simulink library "halout"  (R2021b)
settings: Solver=VariableStepAuto  StartTime=0.0  StopTime=10.0  RelTol=1e-3
undefined symbols (not defined in the file): C_TASK_5MS_S, FALSE, KHAL_CAN1FDAPS3E2E_flg, KHAL_CAN1FDAPS3TxReq_flg, KHAL_CAN1FDVCU2E2E_flg, KHAL_CAN1FDVCU2TxReq_flg, KHAL_CAN1FDVCU3E2E_flg, KHAL_CAN1FDVCU3TxReq_flg, KHAL_CAN1TxReq_flg, KHAL_CAN2TxReq_flg, KHAL_CAN3FDVCU1TxReq_flg, KHAL_CAN3FDVCU2E2E_flg, KHAL_CAN3FDVCU2TxReq_flg, KHAL_CAN3TxReq_flg, KHAL_CAN4FDVCU1E2E_flg, KHAL_CAN4FDVCU1TxReq_flg, KHAL_CAN4TxReq_flg, KHAL_CAN5TxReq_flg, ONE_INT, TRUE, ZERO_INT
libraries: FVT_lib x383, simulink x179
(part 15 of 20)

== system halout/HAL_OUT/CAN2/FD_VCU0_0x1F0/SysAllowReadySta ==
  SysAllowReadySta : Inport
  Data Type Conversion : DataTypeConversion  OutDataTypeStr=uint8  RndMeth=Round
  CAN2_SysAllowReadySta : Outport
  wires:
  Data Type Conversion/1 -> CAN2_SysAllowReadySta/1
  SysAllowReadySta/1 -> Data Type Conversion/1

== system halout/HAL_OUT/CAN2/FD_VCU0_0x1F0/SysPwrSta ==
  SysPwrSta : Inport
  Data Type Conversion : DataTypeConversion  OutDataTypeStr=uint8  RndMeth=Round
  CAN2_SysPwrSta : Outport
  wires:
  Data Type Conversion/1 -> CAN2_SysPwrSta/1
  SysPwrSta/1 -> Data Type Conversion/1

== system halout/HAL_OUT/CAN2/FD_VCU0_0x1F0/TCountSta ==
  TCountSta : Inport
  Data Type Conversion : DataTypeConversion  OutDataTypeStr=uint8  RndMeth=Round
  CAN2_TCountSta : Outport
  wires:
  Data Type Conversion/1 -> CAN2_TCountSta/1
  TCountSta/1 -> Data Type Conversion/1

== system halout/HAL_OUT/CAN2/FD_VCU0_0x1F0/TimerAllowSleep ==
  TimerAllowSleep : Inport
  Data Type Conversion : DataTypeConversion  OutDataTypeStr=uint8  RndMeth=Round
  CAN2_TimerAllowSleep : Outport
  wires:
  Data Type Conversion/1 -> CAN2_TimerAllowSleep/1
  TimerAllowSleep/1 -> Data Type Conversion/1

== system halout/HAL_OUT/CAN2/FD_VCU0_0x1F0/VCUBrkSWSta ==
  VCUBrkSWSta : Inport
  Data Type Conversion : DataTypeConversion  OutDataTypeStr=uint8  RndMeth=Round
  CAN2_VCUBrkSWSta : Outport
  wires:
  Data Type Conversion/1 -> CAN2_VCUBrkSWSta/1
  VCUBrkSWSta/1 -> Data Type Conversion/1

== system halout/HAL_OUT/CAN2/FD_VCU0_0x1F0/VCUFLDoorSta ==
  VCUFLDoorSta : Inport
  Data Type Conversion : DataTypeConversion  OutDataTypeStr=uint8  RndMeth=Round
  CAN2_VCUFLDoorSta : Outport
  wires:
  Data Type Conversion/1 -> CAN2_VCUFLDoorSta/1
  VCUFLDoorSta/1 -> Data Type Conversion/1

== system halout/HAL_OUT/CAN2/FD_VCU0_0x1F0/VCUFRDoorSta ==
  VCUFRDoorSta : Inport
  Data Type Conversion : DataTypeConversion  OutDataTypeStr=uint8  RndMeth=Round
  CAN2_VCUFRDoorSta : Outport
  wires:
  Data Type Conversion/1 -> CAN2_VCUFRDoorSta/1
  VCUFRDoorSta/1 -> Data Type Conversion/1

== system halout/HAL_OUT/CAN2/FD_VCU0_0x1F0/VCUHoodSWSta ==
  VCUHoodSWSta : Inport
  Data Type Conversion : DataTypeConversion  OutDataTypeStr=uint8  RndMeth=Round
  CAN2_VCUHoodSWSta : Outport
  wires:
  Data Type Conversion/1 -> CAN2_VCUHoodSWSta/1
  VCUHoodSWSta/1 -> Data Type Conversion/1

== system halout/HAL_OUT/CAN2/FD_VCU0_0x1F0/VCURLDoorSta ==
  VCURLDoorSta : Inport
  Data Type Conversion : DataTypeConversion  OutDataTypeStr=uint8  RndMeth=Round
  CAN2_VCURLDoorSta : Outport
  wires:
  Data Type Conversion/1 -> CAN2_VCURLDoorSta/1
  VCURLDoorSta/1 -> Data Type Conversion/1

== system halout/HAL_OUT/CAN2/FD_VCU0_0x1F0/VCURRDoorSta ==
  VCURRDoorSta : Inport
  Data Type Conversion : DataTypeConversion  OutDataTypeStr=uint8  RndMeth=Round
  CAN2_VCURRDoorSta : Outport
  wires:
  Data Type Conversion/1 -> CAN2_VCURRDoorSta/1
  VCURRDoorSta/1 -> Data Type Conversion/1

== system halout/HAL_OUT/CAN2/FD_VCU0_0x1F0/VCUTailgateSWSta ==
  VCUTailgateSWSta : Inport
  Data Type Conversion : DataTypeConversion  OutDataTypeStr=uint8  RndMeth=Round
  CAN2_VCUTailgateSWSta : Outport
  wires:
  Data Type Conversion/1 -> CAN2_VCUTailgateSWSta/1
  VCUTailgateSWSta/1 -> Data Type Conversion/1

== system halout/HAL_OUT/CAN2/FD_VCU0_0x1F0/VehHVPwrAvail4THCM ==
  VehHVPwrAvail4THCM : Inport
  Data Type Conversion : DataTypeConversion  OutDataTypeStr=uint8  RndMeth=Round
  convert_out : FVT_lib/hal/convert_out  gain=50  offset=0
  CAN2_VehHVPwrAvail4THCM : Outport
  wires:
  Data Type Conversion/1 -> CAN2_VehHVPwrAvail4THCM/1
  convert_out/1 -> Data Type Conversion/1
  VehHVPwrAvail4THCM/1 -> convert_out/1

== system halout/HAL_OUT/CAN2/FD_VCU1_0x116/ActiveDischReq ==
  ActiveDischReq : Inport
  Data Type Conversion : DataTypeConversion  OutDataTypeStr=uint8  RndMeth=Round
  CAN2_ActiveDischReq : Outport
  wires:
  Data Type Conversion/1 -> CAN2_ActiveDischReq/1
  ActiveDischReq/1 -> Data Type Conversion/1

== system halout/HAL_OUT/CAN2/FD_VCU1_0x116/CCCrlSta ==
  CCCrlSta : Inport
  Data Type Conversion : DataTypeConversion  OutDataTypeStr=uint8  RndMeth=Round
  CAN2_CC_Crl_Sta : Outport
  wires:
  Data Type Conversion/1 -> CAN2_CC_Crl_Sta/1
  CCCrlSta/1 -> Data Type Conversion/1

== system halout/HAL_OUT/CAN2/FD_VCU1_0x116/CSVCU1CAN2 ==
  CSVCU1CAN2 : Inport
  Data Type Conversion : DataTypeConversion  OutDataTypeStr=uint8  RndMeth=Round
  CAN2_CS_VCU1_CAN2 : Outport
  wires:
  Data Type Conversion/1 -> CAN2_CS_VCU1_CAN2/1
  CSVCU1CAN2/1 -> Data Type Conversion/1

== system halout/HAL_OUT/CAN2/FD_VCU1_0x116/CoastDwModeStaChk ==
  CoastDwModeStaChk : Inport
  Data Type Conversion : DataTypeConversion  OutDataTypeStr=uint8  RndMeth=Round
  CAN2_CoastDwModeStaChk : Outport
  wires:
  Data Type Conversion/1 -> CAN2_CoastDwModeStaChk/1
  CoastDwModeStaChk/1 -> Data Type Conversion/1

== system halout/HAL_OUT/CAN2/FD_VCU1_0x116/CreepSWSta ==
  CreepSWSta : Inport
  Data Type Conversion : DataTypeConversion  OutDataTypeStr=uint8  RndMeth=Round
  CAN2_CreepSW_Sta : Outport
  wires:
  Data Type Conversion/1 -> CAN2_CreepSW_Sta/1
  CreepSWSta/1 -> Data Type Conversion/1

== system halout/HAL_OUT/CAN2/FD_VCU1_0x116/DCDCEnaReq ==
  DCDCEnaReq : Inport
  Data Type Conversion : DataTypeConversion  OutDataTypeStr=uint8  RndMeth=Round
  CAN2_DCDCEnaReq : Outport
  wires:
  Data Type Conversion/1 -> CAN2_DCDCEnaReq/1
  DCDCEnaReq/1 -> Data Type Conversion/1

== system halout/HAL_OUT/CAN2/FD_VCU1_0x116/DCDCVoltSetpoint ==
  DCDCVoltSetpoint : Inport
  Data Type Conversion : DataTypeConversion  OutDataTypeStr=uint8  RndMeth=Round
  convert_out : FVT_lib/hal/convert_out  gain=0.0235  offset=12
  CAN2_DCDCVoltSetpoint : Outport
  wires:
  Data Type Conversion/1 -> CAN2_DCDCVoltSetpoint/1
  convert_out/1 -> Data Type Conversion/1
  DCDCVoltSetpoint/1 -> convert_out/1

== system halout/HAL_OUT/CAN2/FD_VCU1_0x116/DemoModeStaChk ==
  DemoModeStaChk : Inport
  Data Type Conversion : DataTypeConversion  OutDataTypeStr=uint8  RndMeth=Round
  CAN2_DemoModeStaChk : Outport
  wires:
  Data Type Conversion/1 -> CAN2_DemoModeStaChk/1
  DemoModeStaChk/1 -> Data Type Conversion/1

== system halout/HAL_OUT/CAN2/FD_VCU1_0x116/DisengagePFail ==
  DisengagePFail : Inport
  Data Type Conversion : DataTypeConversion  OutDataTypeStr=uint8  RndMeth=Round
  CAN2_DisengageP_Fail : Outport
  wires:
  Data Type Conversion/1 -> CAN2_DisengageP_Fail/1
  DisengagePFail/1 -> Data Type Conversion/1

== system halout/HAL_OUT/CAN2/FD_VCU1_0x116/DrSeatSta ==
  DrSeatSta : Inport
  Data Type Conversion : DataTypeConversion  OutDataTypeStr=uint8  RndMeth=Round
  CAN2_Dr_SeatSta : Outport
  wires:
  Data Type Conversion/1 -> CAN2_Dr_SeatSta/1
  DrSeatSta/1 -> Data Type Conversion/1

== system halout/HAL_OUT/CAN2/FD_VCU1_0x116/DynoModeStaChk ==
  DynoModeStaChk : Inport
  Data Type Conversion : DataTypeConversion  OutDataTypeStr=uint8  RndMeth=Round
  CAN2_DynoModeStaChk : Outport
  wires:
  Data Type Conversion/1 -> CAN2_DynoModeStaChk/1
  DynoModeStaChk/1 -> Data Type Conversion/1

== system halout/HAL_OUT/CAN2/FD_VCU1_0x116/EngagePFail ==
  EngagePFail : Inport
  Data Type Conversion : DataTypeConversion  OutDataTypeStr=uint8  RndMeth=Round
  CAN2_EngageP_Fail : Outport
  wires:
  Data Type Conversion/1 -> CAN2_EngageP_Fail/1
  EngagePFail/1 -> Data Type Conversion/1

== system halout/HAL_OUT/CAN2/FD_VCU1_0x116/FDCVCUPwrSaveReqCmd ==
  FDCVCUPwrSaveReqCmd : Inport
  Data Type Conversion : DataTypeConversion  OutDataTypeStr=uint8  RndMeth=Round
  CAN2_FDC_VCU_PwrSaveReq_Cmd : Outport
  wires:
  Data Type Conversion/1 -> CAN2_FDC_VCU_PwrSaveReq_Cmd/1
  FDCVCUPwrSaveReqCmd/1 -> Data Type Conversion/1

== system halout/HAL_OUT/CAN2/FD_VCU1_0x116/FalseNPreventSta ==
  FalseNPreventSta : Inport
  Data Type Conversion : DataTypeConversion  OutDataTypeStr=uint8  RndMeth=Round
  CAN2_FalseNPrevent_Sta : Outport
  wires:
  Data Type Conversion/1 -> CAN2_FalseNPrevent_Sta/1
  FalseNPreventSta/1 -> Data Type Conversion/1

== system halout/HAL_OUT/CAN2/FD_VCU1_0x116/FrActvDmpDisabReq ==
  FrActvDmpDisabReq : Inport
  Data Type Conversion : DataTypeConversion  OutDataTypeStr=uint8  RndMeth=Round
  CAN2_Fr_ActvDmpDisabReq : Outport
  wires:
  Data Type Conversion/1 -> CAN2_Fr_ActvDmpDisabReq/1
  FrActvDmpDisabReq/1 -> Data Type Conversion/1

== system halout/HAL_OUT/CAN2/FD_VCU1_0x116/FrMCUEnaReq ==
  FrMCUEnaReq : Inport
  Data Type Conversion : DataTypeConversion  OutDataTypeStr=uint8  RndMeth=Round
  CAN2_Fr_MCUEnaReq : Outport
  wires:
  Data Type Conversion/1 -> CAN2_Fr_MCUEnaReq/1
  FrMCUEnaReq/1 -> Data Type Conversion/1

== system halout/HAL_OUT/CAN2/FD_VCU1_0x116/HVBatCnctReq ==
  HVBatCnctReq : Inport
  Data Type Conversion : DataTypeConversion  OutDataTypeStr=uint8  RndMeth=Round
  CAN2_HVBatCnctReq : Outport
  wires:
  Data Type Conversion/1 -> CAN2_HVBatCnctReq/1
  HVBatCnctReq/1 -> Data Type Conversion/1

== system halout/HAL_OUT/CAN2/FD_VCU1_0x116/HVSysReadyToCharge ==
  HVSysReadyToCharge : Inport
  Data Type Conversion : DataTypeConversion  OutDataTypeStr=uint8  RndMeth=Round
  CAN2_HVSysReadyToCharge : Outport
  wires:
  Data Type Conversion/1 -> CAN2_HVSysReadyToCharge/1
  HVSysReadyToCharge/1 -> Data Type Conversion/1

== system halout/HAL_OUT/CAN2/FD_VCU1_0x116/LVChrgFuncStaChk ==
  LVChrgFuncStaChk : Inport
  Data Type Conversion : DataTypeConversion  OutDataTypeStr=uint8  RndMeth=Round
  CAN2_LVChrgFuncStaChk : Outport
  wires:
  Data Type Conversion/1 -> CAN2_LVChrgFuncStaChk/1
  LVChrgFuncStaChk/1 -> Data Type Conversion/1

== system halout/HAL_OUT/CAN2/FD_VCU1_0x116/MSACrlSta ==
  MSACrlSta : Inport
  Data Type Conversion : DataTypeConversion  OutDataTypeStr=uint8  RndMeth=Round
  CAN2_MSA_Crl_Sta : Outport
  wires:
  Data Type Conversion/1 -> CAN2_MSA_Crl_Sta/1
  MSACrlSta/1 -> Data Type Conversion/1

== system halout/HAL_OUT/CAN2/FD_VCU1_0x116/PrkReq ==
  PrkReq : Inport
  Data Type Conversion : DataTypeConversion  OutDataTypeStr=uint8  RndMeth=Round
  CAN2_PrkReq : Outport
  wires:
  Data Type Conversion/1 -> CAN2_PrkReq/1
  PrkReq/1 -> Data Type Conversion/1

== system halout/HAL_OUT/CAN2/FD_VCU1_0x116/PwrSta ==
  PwrSta : Inport
  Data Type Conversion : DataTypeConversion  OutDataTypeStr=uint8  RndMeth=Round
  CAN2_PwrSta : Outport
  wires:
  Data Type Conversion/1 -> CAN2_PwrSta/1
  PwrSta/1 -> Data Type Conversion/1

== system halout/HAL_OUT/CAN2/FD_VCU1_0x116/RCVCU1CAN2 ==
  RCVCU1CAN2 : Inport
  Data Type Conversion : DataTypeConversion  OutDataTypeStr=uint8  RndMeth=Round
  CAN2_RC_VCU1_CAN2 : Outport
  wires:
  Data Type Conversion/1 -> CAN2_RC_VCU1_CAN2/1
  RCVCU1CAN2/1 -> Data Type Conversion/1

== system halout/HAL_OUT/CAN2/FD_VCU1_0x116/RrActvDmpDisabReq ==
  RrActvDmpDisabReq : Inport
  Data Type Conversion : DataTypeConversion  OutDataTypeStr=uint8  RndMeth=Round
  CAN2_Rr_ActvDmpDisabReq : Outport
  wires:
  Data Type Conversion/1 -> CAN2_Rr_ActvDmpDisabReq/1
  RrActvDmpDisabReq/1 -> Data Type Conversion/1

== system halout/HAL_OUT/CAN2/FD_VCU1_0x116/RrMCUEnaReq ==
  RrMCUEnaReq : Inport
  Data Type Conversion : DataTypeConversion  OutDataTypeStr=uint8  RndMeth=Round
  CAN2_Rr_MCUEnaReq : Outport
  wires:
  Data Type Conversion/1 -> CAN2_Rr_MCUEnaReq/1
  RrMCUEnaReq/1 -> Data Type Conversion/1

== system halout/HAL_OUT/CAN2/FD_VCU1_0x116/ShiftGearPosn ==
  ShiftGearPosn : Inport
  Data Type Conversion : DataTypeConversion  OutDataTypeStr=uint8  RndMeth=Round
  CAN2_ShiftGearPosn : Outport
  wires:
  Data Type Conversion/1 -> CAN2_ShiftGearPosn/1
  ShiftGearPosn/1 -> Data Type Conversion/1

== system halout/HAL_OUT/CAN2/FD_VCU1_0x116/VCUOPDHold ==
  VCUOPDHold : Inport
  Data Type Conversion : DataTypeConversion  OutDataTypeStr=uint8  RndMeth=Round
  CAN2_VCU_OPDHold : Outport
  wires:
  Data Type Conversion/1 -> CAN2_VCU_OPDHold/1
  VCUOPDHold/1 -> Data Type Conversion/1

== system halout/HAL_OUT/CAN2/FD_VCU1_0x116/XWDMode ==
  XWDMode : Inport
  Data Type Conversion : DataTypeConversion  OutDataTypeStr=uint8  RndMeth=Round
  CAN2_XWDMode : Outport
  wires:
  Data Type Conversion/1 -> CAN2_XWDMode/1
  XWDMode/1 -> Data Type Conversion/1

== system halout/HAL_OUT/CAN2/FD_VCU2_0x154/ACCCtrlAvail ==
  ACCCtrlAvail : Inport
  Data Type Conversion : DataTypeConversion  OutDataTypeStr=uint8  RndMeth=Round
  CAN2_ACC_CtrlAvail : Outport
  wires:
  Data Type Conversion/1 -> CAN2_ACC_CtrlAvail/1
  ACCCtrlAvail/1 -> Data Type Conversion/1

== system halout/HAL_OUT/CAN2/FD_VCU2_0x154/AccPedalOverride ==
  AccPedalOverride : Inport
  Data Type Conversion : DataTypeConversion  OutDataTypeStr=uint8  RndMeth=Round
  CAN2_AccPedal_Override : Outport
  wires:
  Data Type Conversion/1 -> CAN2_AccPedal_Override/1
  AccPedalOverride/1 -> Data Type Conversion/1

== system halout/HAL_OUT/CAN2/FD_VCU2_0x154/ActAPSPosn ==
  ActAPSPosn : Inport
  Data Type Conversion : DataTypeConversion  OutDataTypeStr=uint8  RndMeth=Round
  convert_out : FVT_lib/hal/convert_out  gain=0.394  offset=0
  CAN2_ActAPSPosn : Outport
  wires:
  Data Type Conversion/1 -> CAN2_ActAPSPosn/1
  convert_out/1 -> Data Type Conversion/1
  ActAPSPosn/1 -> convert_out/1

== system halout/HAL_OUT/CAN2/FD_VCU2_0x154/CSVCU2CAN1 ==
  CSVCU2CAN1 : Inport
  Data Type Conversion : DataTypeConversion  OutDataTypeStr=uint8  RndMeth=Round
  CAN2_CS_VCU2_CAN1 : Outport
  wires:
  Data Type Conversion/1 -> CAN2_CS_VCU2_CAN1/1
  CSVCU2CAN1/1 -> Data Type Conversion/1

== system halout/HAL_OUT/CAN2/FD_VCU2_0x154/DriverTq ==
  DriverTq : Inport
  Data Type Conversion : DataTypeConversion  OutDataTypeStr=uint16  RndMeth=Round
  convert_out : FVT_lib/hal/convert_out  gain=1  offset=-4300
  CAN2_DriverTq : Outport
  wires:
  Data Type Conversion/1 -> CAN2_DriverTq/1
  convert_out/1 -> Data Type Conversion/1
  DriverTq/1 -> convert_out/1

== system halout/HAL_OUT/CAN2/FD_VCU2_0x154/FrDriverTq ==
  FrDriverTq : Inport
  Data Type Conversion : DataTypeConversion  OutDataTypeStr=uint16  RndMeth=Round
  convert_out : FVT_lib/hal/convert_out  gain=0.5  offset=-5300
  CAN2_Fr_DriverTq : Outport
  wires:
  Data Type Conversion/1 -> CAN2_Fr_DriverTq/1
  convert_out/1 -> Data Type Conversion/1
  FrDriverTq/1 -> convert_out/1

== system halout/HAL_OUT/CAN2/FD_VCU2_0x154/RCVCU2CAN1 ==
  RCVCU2CAN1 : Inport
  Data Type Conversion : DataTypeConversion  OutDataTypeStr=uint8  RndMeth=Round
  CAN2_RC_VCU2_CAN1 : Outport
  wires:
  Data Type Conversion/1 -> CAN2_RC_VCU2_CAN1/1
  RCVCU2CAN1/1 -> Data Type Conversion/1

== system halout/HAL_OUT/CAN2/FD_VCU2_0x154/RrDriverTq ==
  RrDriverTq : Inport
  Data Type Conversion : DataTypeConversion  OutDataTypeStr=uint16  RndMeth=Round
  convert_out : FVT_lib/hal/convert_out  gain=0.5  offset=-5300
  CAN2_Rr_DriverTq : Outport
  wires:
  Data Type Conversion/1 -> CAN2_Rr_DriverTq/1
  convert_out/1 -> Data Type Conversion/1
  RrDriverTq/1 -> convert_out/1

== system halout/HAL_OUT/CAN2/FD_VCU2_0x154/VehActPwr ==
  VehActPwr : Inport
  Data Type Conversion : DataTypeConversion  OutDataTypeStr=uint32  RndMeth=Round
  convert_out : FVT_lib/hal/convert_out  gain=1  offset=-600000
  CAN2_VehActPwr : Outport
  wires:
  Data Type Conversion/1 -> CAN2_VehActPwr/1
  convert_out/1 -> Data Type Conversion/1
  VehActPwr/1 -> convert_out/1

== system halout/HAL_OUT/CAN2/FD_VCU4_0x3C0/EVDriveMode ==
  EVDriveMode : Inport
  Data Type Conversion : DataTypeConversion  OutDataTypeStr=uint8  RndMeth=Round
  CAN2_EVDriveMode : Outport
  wires:
  Data Type Conversion/1 -> CAN2_EVDriveMode/1
  EVDriveMode/1 -> Data Type Conversion/1

== system halout/HAL_OUT/CAN2/FD_VCU4_0x3C0/EngAGSCloseSta ==
  EngAGSCloseSta : Inport
  Data Type Conversion : DataTypeConversion  OutDataTypeStr=uint8  RndMeth=Round
  CAN2_Eng_AGSCloseSta : Outport
  wires:
  Data Type Conversion/1 -> CAN2_Eng_AGSCloseSta/1
  EngAGSCloseSta/1 -> Data Type Conversion/1

== system halout/HAL_OUT/CAN2/FD_VCU4_0x3C0/EngActvDmpDisabSta ==
  EngActvDmpDisabSta : Inport
  Data Type Conversion : DataTypeConversion  OutDataTypeStr=uint8  RndMeth=Round
  CAN2_Eng_ActvDmpDisabSta : Outport
  wires:
  Data Type Conversion/1 -> CAN2_Eng_ActvDmpDisabSta/1
  EngActvDmpDisabSta/1 -> Data Type Conversion/1

== system halout/HAL_OUT/CAN2/FD_VCU4_0x3C0/EngCoastDwSta ==
  EngCoastDwSta : Inport
  Data Type Conversion : DataTypeConversion  OutDataTypeStr=uint8  RndMeth=Round
  CAN2_Eng_CoastDwSta : Outport
  wires:
  Data Type Conversion/1 -> CAN2_Eng_CoastDwSta/1
  EngCoastDwSta/1 -> Data Type Conversion/1

== system halout/HAL_OUT/CAN2/FD_VCU4_0x3C0/EngPwrLockSta ==
  EngPwrLockSta : Inport
  Data Type Conversion : DataTypeConversion  OutDataTypeStr=uint8  RndMeth=Round
  CAN2_Eng_PwrLockSta : Outport
  wires:
  Data Type Conversion/1 -> CAN2_Eng_PwrLockSta/1
  EngPwrLockSta/1 -> Data Type Conversion/1

== system halout/HAL_OUT/CAN2/FD_VCU4_0x3C0/VCUACCErr ==
  VCUACCErr : Inport
  Data Type Conversion : DataTypeConversion  OutDataTypeStr=uint8  RndMeth=Round
  CAN2_VCU_ACCErr : Outport
  wires:
  Data Type Conversion/1 -> CAN2_VCU_ACCErr/1
  VCUACCErr/1 -> Data Type Conversion/1

== system halout/HAL_OUT/CAN2/FD_VCU4_0x3C0/VCUISAErr ==
  VCUISAErr : Inport
  Data Type Conversion : DataTypeConversion  OutDataTypeStr=uint8  RndMeth=Round
  CAN2_VCU_ISAErr : Outport
  wires:
  Data Type Conversion/1 -> CAN2_VCU_ISAErr/1
  VCUISAErr/1 -> Data Type Conversion/1

== system halout/HAL_OUT/CAN2/FD_VCU4_0x3C0/VehMalfunLevel ==
  VehMalfunLevel : Inport
  Data Type Conversion : DataTypeConversion  OutDataTypeStr=uint8  RndMeth=Round
  CAN2_VehMalfunLevel : Outport
  wires:
  Data Type Conversion/1 -> CAN2_VehMalfunLevel/1
  VehMalfunLevel/1 -> Data Type Conversion/1

== system halout/HAL_OUT/CAN2/FD_VCU4_0x3C0/ZoneDRSCPCommErr ==
  ZoneDRSCPCommErr : Inport
  Data Type Conversion : DataTypeConversion  OutDataTypeStr=uint8  RndMeth=Round
  CAN2_ZoneDR_SCP_CommErr : Outport
  wires:
  Data Type Conversion/1 -> CAN2_ZoneDR_SCP_CommErr/1
  ZoneDRSCPCommErr/1 -> Data Type Conversion/1

== system halout/HAL_OUT/CAN2/FD_VCU5_0x245/EDriveSysErrAccPedalErr ==
  EDriveSysErrAccPedalErr : Inport
  Data Type Conversion : DataTypeConversion  OutDataTypeStr=uint8  RndMeth=Round
  CAN2_EDriveSysErr_AccPedalErr : Outport
  wires:
  Data Type Conversion/1 -> CAN2_EDriveSysErr_AccPedalErr/1
  EDriveSysErrAccPedalErr/1 -> Data Type Conversion/1

== system halout/HAL_OUT/CAN2/FD_VCU5_0x245/EDriveSysErrMCUErr ==
  EDriveSysErrMCUErr : Inport
  Data Type Conversion : DataTypeConversion  OutDataTypeStr=uint8  RndMeth=Round
  CAN2_EDriveSysErr_MCUErr : Outport
  wires:
  Data Type Conversion/1 -> CAN2_EDriveSysErr_MCUErr/1
  EDriveSysErrMCUErr/1 -> Data Type Conversion/1

== system halout/HAL_OUT/CAN2/FD_VCU5_0x245/EDriveSysErrShifterErr ==
  EDriveSysErrShifterErr : Inport
  Data Type Conversion : DataTypeConversion  OutDataTypeStr=uint8  RndMeth=Round
  CAN2_EDriveSysErr_ShifterErr : Outport
  wires:
  Data Type Conversion/1 -> CAN2_EDriveSysErr_ShifterErr/1
  EDriveSysErrShifterErr/1 -> Data Type Conversion/1

== system halout/HAL_OUT/CAN2/FD_VCU5_0x245/EDriveSysErrVCUErr ==
  EDriveSysErrVCUErr : Inport
  Data Type Conversion : DataTypeConversion  OutDataTypeStr=uint8  RndMeth=Round
  CAN2_EDriveSysErr_VCUErr : Outport
  wires:
  Data Type Conversion/1 -> CAN2_EDriveSysErr_VCUErr/1
  EDriveSysErrVCUErr/1 -> Data Type Conversion/1

== system halout/HAL_OUT/CAN2/FD_VCU5_0x245/HVSysErrIsolationErr ==
  HVSysErrIsolationErr : Inport
  Data Type Conversion : DataTypeConversion  OutDataTypeStr=uint8  RndMeth=Round
  CAN2_HVSysErr_IsolationErr : Outport
  wires:
  Data Type Conversion/1 -> CAN2_HVSysErr_IsolationErr/1
  HVSysErrIsolationErr/1 -> Data Type Conversion/1

== system halout/HAL_OUT/CAN2/FD_VCU5_0x245/HVSysErrPackErr ==
  HVSysErrPackErr : Inport
  Data Type Conversion : DataTypeConversion  OutDataTypeStr=uint8  RndMeth=Round
  CAN2_HVSysErr_PackErr : Outport
  wires:
  Data Type Conversion/1 -> CAN2_HVSysErr_PackErr/1
  HVSysErrPackErr/1 -> Data Type Conversion/1

== system halout/HAL_OUT/CAN2/FD_VCU5_0x245/HVSysErrRelayErr ==
  HVSysErrRelayErr : Inport
  Data Type Conversion : DataTypeConversion  OutDataTypeStr=uint8  RndMeth=Round
  CAN2_HVSysErr_RelayErr : Outport
  wires:
  Data Type Conversion/1 -> CAN2_HVSysErr_RelayErr/1
  HVSysErrRelayErr/1 -> Data Type Conversion/1

== system halout/HAL_OUT/CAN2/FD_VCU5_0x245/LVSysErrPwrOutpErr ==
  LVSysErrPwrOutpErr : Inport
  Data Type Conversion : DataTypeConversion  OutDataTypeStr=uint8  RndMeth=Round
  CAN2_LVSysErr_PwrOutpErr : Outport
  wires:
  Data Type Conversion/1 -> CAN2_LVSysErr_PwrOutpErr/1
  LVSysErrPwrOutpErr/1 -> Data Type Conversion/1

== system halout/HAL_OUT/CAN2/FD_VCU5_0x245/LimphomeAct ==
  LimphomeAct : Inport
  Data Type Conversion : DataTypeConversion  OutDataTypeStr=uint8  RndMeth=Round
  CAN2_LimphomeAct : Outport
  wires:
  Data Type Conversion/1 -> CAN2_LimphomeAct/1
  LimphomeAct/1 -> Data Type Conversion/1

== system halout/HAL_OUT/CAN2/FD_VCU5_0x245/LowSOCWarn ==
  LowSOCWarn : Inport
  Data Type Conversion : DataTypeConversion  OutDataTypeStr=uint8  RndMeth=Round
  CAN2_LowSOCWarn : Outport
  wires:
  Data Type Conversion/1 -> CAN2_LowSOCWarn/1
  LowSOCWarn/1 -> Data Type Conversion/1

== system halout/HAL_OUT/CAN2/FD_VCU5_0x245/PwrStaErr ==
  PwrStaErr : Inport
  Data Type Conversion : DataTypeConversion  OutDataTypeStr=uint8  RndMeth=Round
  CAN2_PwrStaErr : Outport
  wires:
  Data Type Conversion/1 -> CAN2_PwrStaErr/1
  PwrStaErr/1 -> Data Type Conversion/1

== system halout/HAL_OUT/CAN2/FD_VCU5_0x245/ReVehThdChkSta ==
  ReVehThdChkSta : Inport
  Data Type Conversion : DataTypeConversion  OutDataTypeStr=uint8  RndMeth=Round
  CAN2_Re_VehThdChkSta : Outport
  wires:
  Data Type Conversion/1 -> CAN2_Re_VehThdChkSta/1
  ReVehThdChkSta/1 -> Data Type Conversion/1

== system halout/HAL_OUT/CAN2/FD_VCU6_0x3C3/FUSIONHWVer1 ==
  FUSIONHWVer1 : Inport
  Data Type Conversion : DataTypeConversion  OutDataTypeStr=uint8  RndMeth=Round
  CAN2_FUSION_HW_Ver1 : Outport
  wires:
  Data Type Conversion/1 -> CAN2_FUSION_HW_Ver1/1
  FUSIONHWVer1/1 -> Data Type Conversion/1

== system halout/HAL_OUT/CAN2/FD_VCU6_0x3C3/FUSIONHWVer2 ==
  FUSIONHWVer2 : Inport
  Data Type Conversion : DataTypeConversion  OutDataTypeStr=uint8  RndMeth=Round
  CAN2_FUSION_HW_Ver2 : Outport
  wires:
  Data Type Conversion/1 -> CAN2_FUSION_HW_Ver2/1
  FUSIONHWVer2/1 -> Data Type Conversion/1

== system halout/HAL_OUT/CAN2/FD_VCU6_0x3C3/FUSIONHWVer3 ==
  FUSIONHWVer3 : Inport
  Data Type Conversion : DataTypeConversion  OutDataTypeStr=uint8  RndMeth=Round
  CAN2_FUSION_HW_Ver3 : Outport
  wires:
  Data Type Conversion/1 -> CAN2_FUSION_HW_Ver3/1
  FUSIONHWVer3/1 -> Data Type Conversion/1

== system halout/HAL_OUT/CAN2/FD_VCU6_0x3C3/FUSIONSWCarModel1 ==
  FUSIONSWCarModel1 : Inport
  Data Type Conversion : DataTypeConversion  OutDataTypeStr=uint8  RndMeth=Round
  CAN2_FUSION_SW_CarModel1 : Outport
  wires:
  Data Type Conversion/1 -> CAN2_FUSION_SW_CarModel1/1
  FUSIONSWCarModel1/1 -> Data Type Conversion/1

== system halout/HAL_OUT/CAN2/FD_VCU6_0x3C3/FUSIONSWCarModel2 ==
  FUSIONSWCarModel2 : Inport
  Data Type Conversion : DataTypeConversion  OutDataTypeStr=uint8  RndMeth=Round
  CAN2_FUSION_SW_CarModel2 : Outport
  wires:
  Data Type Conversion/1 -> CAN2_FUSION_SW_CarModel2/1
  FUSIONSWCarModel2/1 -> Data Type Conversion/1

== system halout/HAL_OUT/CAN2/FD_VCU6_0x3C3/FUSIONSWCarModel3 ==
  FUSIONSWCarModel3 : Inport
  Data Type Conversion : DataTypeConversion  OutDataTypeStr=uint8  RndMeth=Round
  CAN2_FUSION_SW_CarModel3 : Outport
  wires:
  Data Type Conversion/1 -> CAN2_FUSION_SW_CarModel3/1
  FUSIONSWCarModel3/1 -> Data Type Conversion/1

== system halout/HAL_OUT/CAN2/FD_VCU6_0x3C3/FUSIONSWController1 ==
  FUSIONSWController1 : Inport
  Data Type Conversion : DataTypeConversion  OutDataTypeStr=uint8  RndMeth=Round
  CAN2_FUSION_SW_Controller1 : Outport
  wires:
  Data Type Conversion/1 -> CAN2_FUSION_SW_Controller1/1
  FUSIONSWController1/1 -> Data Type Conversion/1

== system halout/HAL_OUT/CAN2/FD_VCU6_0x3C3/FUSIONSWController2 ==
  FUSIONSWController2 : Inport
  Data Type Conversion : DataTypeConversion  OutDataTypeStr=uint8  RndMeth=Round
  CAN2_FUSION_SW_Controller2 : Outport
  wires:
  Data Type Conversion/1 -> CAN2_FUSION_SW_Controller2/1
  FUSIONSWController2/1 -> Data Type Conversion/1

== system halout/HAL_OUT/CAN2/FD_VCU6_0x3C3/FUSIONSWCountry1 ==
  FUSIONSWCountry1 : Inport
  Data Type Conversion : DataTypeConversion  OutDataTypeStr=uint8  RndMeth=Round
  CAN2_FUSION_SW_Country1 : Outport
  wires:
  Data Type Conversion/1 -> CAN2_FUSION_SW_Country1/1
  FUSIONSWCountry1/1 -> Data Type Conversion/1

== system halout/HAL_OUT/CAN2/FD_VCU6_0x3C3/FUSIONSWCountry2 ==
  FUSIONSWCountry2 : Inport
  Data Type Conversion : DataTypeConversion  OutDataTypeStr=uint8  RndMeth=Round
  CAN2_FUSION_SW_Country2 : Outport
  wires:
  Data Type Conversion/1 -> CAN2_FUSION_SW_Country2/1
  FUSIONSWCountry2/1 -> Data Type Conversion/1

== system halout/HAL_OUT/CAN2/FD_VCU6_0x3C3/FUSIONSWMajor1 ==
  FUSIONSWMajor1 : Inport
  Data Type Conversion : DataTypeConversion  OutDataTypeStr=uint8  RndMeth=Round
  CAN2_FUSION_SW_Major1 : Outport
  wires:
  Data Type Conversion/1 -> CAN2_FUSION_SW_Major1/1
  FUSIONSWMajor1/1 -> Data Type Conversion/1

== system halout/HAL_OUT/CAN2/FD_VCU6_0x3C3/FUSIONSWMajor2 ==
  FUSIONSWMajor2 : Inport
  Data Type Conversion : DataTypeConversion  OutDataTypeStr=uint8  RndMeth=Round
  CAN2_FUSION_SW_Major2 : Outport
  wires:
  Data Type Conversion/1 -> CAN2_FUSION_SW_Major2/1
  FUSIONSWMajor2/1 -> Data Type Conversion/1

== system halout/HAL_OUT/CAN2/FD_VCU6_0x3C3/FUSIONSWMinor1 ==
  FUSIONSWMinor1 : Inport
  Data Type Conversion : DataTypeConversion  OutDataTypeStr=uint8  RndMeth=Round
  CAN2_FUSION_SW_Minor1 : Outport
  wires:
  Data Type Conversion/1 -> CAN2_FUSION_SW_Minor1/1
  FUSIONSWMinor1/1 -> Data Type Conversion/1

== system halout/HAL_OUT/CAN2/FD_VCU6_0x3C3/FUSIONSWMinor2 ==
  FUSIONSWMinor2 : Inport
  Data Type Conversion : DataTypeConversion  OutDataTypeStr=uint8  RndMeth=Round
  CAN2_FUSION_SW_Minor2 : Outport
  wires:
  Data Type Conversion/1 -> CAN2_FUSION_SW_Minor2/1
  FUSIONSWMinor2/1 -> Data Type Conversion/1

== system halout/HAL_OUT/CAN2/FD_VCU6_0x3C3/FUSIONSWPatch1 ==
  FUSIONSWPatch1 : Inport
  Data Type Conversion : DataTypeConversion  OutDataTypeStr=uint8  RndMeth=Round
  CAN2_FUSION_SW_Patch1 : Outport
  wires:
  Data Type Conversion/1 -> CAN2_FUSION_SW_Patch1/1
  FUSIONSWPatch1/1 -> Data Type Conversion/1

== system halout/HAL_OUT/CAN2/FD_VCU6_0x3C3/FUSIONSWPatch2 ==
  FUSIONSWPatch2 : Inport
  Data Type Conversion : DataTypeConversion  OutDataTypeStr=uint8  RndMeth=Round
  CAN2_FUSION_SW_Patch2 : Outport
  wires:
  Data Type Conversion/1 -> CAN2_FUSION_SW_Patch2/1
  FUSIONSWPatch2/1 -> Data Type Conversion/1

== system halout/HAL_OUT/CAN2/FD_VCU6_0x3C3/FUSIONSWSHA1 ==
  FUSIONSWSHA1 : Inport
  Data Type Conversion : DataTypeConversion  OutDataTypeStr=uint8  RndMeth=Round
  CAN2_FUSION_SW_SHA1 : Outport
  wires:
  Data Type Conversion/1 -> CAN2_FUSION_SW_SHA1/1
  FUSIONSWSHA1/1 -> Data Type Conversion/1

== system halout/HAL_OUT/CAN2/FD_VCU6_0x3C3/FUSIONSWSHA2 ==
  FUSIONSWSHA2 : Inport
  Data Type Conversion : DataTypeConversion  OutDataTypeStr=uint8  RndMeth=Round
  CAN2_FUSION_SW_SHA2 : Outport
  wires:
  Data Type Conversion/1 -> CAN2_FUSION_SW_SHA2/1
  FUSIONSWSHA2/1 -> Data Type Conversion/1

== system halout/HAL_OUT/CAN2/FD_VCU6_0x3C3/FUSIONSWSHA3 ==
  FUSIONSWSHA3 : Inport
  Data Type Conversion : DataTypeConversion  OutDataTypeStr=uint8  RndMeth=Round
  CAN2_FUSION_SW_SHA3 : Outport
  wires:
  Data Type Conversion/1 -> CAN2_FUSION_SW_SHA3/1
  FUSIONSWSHA3/1 -> Data Type Conversion/1

== system halout/HAL_OUT/CAN2/FD_VCU6_0x3C3/FUSIONSWSHA4 ==
  FUSIONSWSHA4 : Inport
  Data Type Conversion : DataTypeConversion  OutDataTypeStr=uint8  RndMeth=Round
  CAN2_FUSION_SW_SHA4 : Outport
  wires:
  Data Type Conversion/1 -> CAN2_FUSION_SW_SHA4/1
  FUSIONSWSHA4/1 -> Data Type Conversion/1

== system halout/HAL_OUT/CAN2/FD_VCU6_0x3C3/FUSIONSWSHA5 ==
  FUSIONSWSHA5 : Inport
  Data Type Conversion : DataTypeConversion  OutDataTypeStr=uint8  RndMeth=Round
  CAN2_FUSION_SW_SHA5 : Outport
  wires:
  Data Type Conversion/1 -> CAN2_FUSION_SW_SHA5/1
  FUSIONSWSHA5/1 -> Data Type Conversion/1

== system halout/HAL_OUT/CAN2/FD_VCU6_0x3C3/FUSIONSWSHA6 ==
  FUSIONSWSHA6 : Inport
  Data Type Conversion : DataTypeConversion  OutDataTypeStr=uint8  RndMeth=Round
  CAN2_FUSION_SW_SHA6 : Outport
  wires:
  Data Type Conversion/1 -> CAN2_FUSION_SW_SHA6/1
  FUSIONSWSHA6/1 -> Data Type Conversion/1

== system halout/HAL_OUT/CAN2/FD_VCU6_0x3C3/FUSIONSWSHA7 ==
  FUSIONSWSHA7 : Inport
  Data Type Conversion : DataTypeConversion  OutDataTypeStr=uint8  RndMeth=Round
  CAN2_FUSION_SW_SHA7 : Outport
  wires:
  Data Type Conversion/1 -> CAN2_FUSION_SW_SHA7/1
  FUSIONSWSHA7/1 -> Data Type Conversion/1

== system halout/HAL_OUT/CAN2/FD_VCU6_0x3C3/FUSIONSWSHA8 ==
  FUSIONSWSHA8 : Inport
  Data Type Conversion : DataTypeConversion  OutDataTypeStr=uint8  RndMeth=Round
  CAN2_FUSION_SW_SHA8 : Outport
  wires:
  Data Type Conversion/1 -> CAN2_FUSION_SW_SHA8/1
  FUSIONSWSHA8/1 -> Data Type Conversion/1

== system halout/HAL_OUT/CAN2/FD_VCU6_0x3C3/FUSIONSWVar ==
  FUSIONSWVar : Inport
  Data Type Conversion : DataTypeConversion  OutDataTypeStr=uint8  RndMeth=Round
  CAN2_FUSION_SW_Var : Outport
  wires:
  Data Type Conversion/1 -> CAN2_FUSION_SW_Var/1
  FUSIONSWVar/1 -> Data Type Conversion/1

== system halout/HAL_OUT/CAN2/FD_VCU6_0x3C3/FUSIONSWchange1 ==
  FUSIONSWchange1 : Inport
  Data Type Conversion : DataTypeConversion  OutDataTypeStr=uint8  RndMeth=Round
  CAN2_FUSION_SW_change1 : Outport
  wires:
  Data Type Conversion/1 -> CAN2_FUSION_SW_change1/1
  FUSIONSWchange1/1 -> Data Type Conversion/1

== system halout/HAL_OUT/CAN2/FD_VCU6_0x3C3/FUSIONSWchange2 ==
  FUSIONSWchange2 : Inport
  Data Type Conversion : DataTypeConversion  OutDataTypeStr=uint8  RndMeth=Round
  CAN2_FUSION_SW_change2 : Outport
  wires:
  Data Type Conversion/1 -> CAN2_FUSION_SW_change2/1
  FUSIONSWchange2/1 -> Data Type Conversion/1

== system halout/HAL_OUT/CAN2/FD_VCU6_0x3C3/FUSIONSWdash1 ==
  FUSIONSWdash1 : Inport
  Data Type Conversion : DataTypeConversion  OutDataTypeStr=uint8  RndMeth=Round
  CAN2_FUSION_SW_dash1 : Outport
  wires:
  Data Type Conversion/1 -> CAN2_FUSION_SW_dash1/1
  FUSIONSWdash1/1 -> Data Type Conversion/1

== system halout/HAL_OUT/CAN2/FD_VCU6_0x3C3/FUSIONSWdash2 ==
  FUSIONSWdash2 : Inport
  Data Type Conversion : DataTypeConversion  OutDataTypeStr=uint8  RndMeth=Round
  CAN2_FUSION_SW_dash2 : Outport
  wires:
  Data Type Conversion/1 -> CAN2_FUSION_SW_dash2/1
  FUSIONSWdash2/1 -> Data Type Conversion/1

== system halout/HAL_OUT/CAN2/FD_VMC1_0x17F/CCMSASpdWar ==
  CCMSASpdWar : Inport
  Data Type Conversion : DataTypeConversion  OutDataTypeStr=uint8  RndMeth=Round
  CAN2_CCMSA_SpdWar : Outport
  wires:
  Data Type Conversion/1 -> CAN2_CCMSA_SpdWar/1
  CCMSASpdWar/1 -> Data Type Conversion/1

== system halout/HAL_OUT/CAN3/FD_BCM1_0x216/AllDoorSW ==
  AllDoorSW : Inport
  Data Type Conversion : DataTypeConversion  OutDataTypeStr=uint8  RndMeth=Round
  CAN3_AllDoorSW : Outport
  wires:
  Data Type Conversion/1 -> CAN3_AllDoorSW/1
  AllDoorSW/1 -> Data Type Conversion/1

== system halout/HAL_OUT/CAN3/FD_BCM1_0x216/AntiTheftSeatFold ==
  AntiTheftSeatFold : Inport
  Data Type Conversion : DataTypeConversion  OutDataTypeStr=uint8  RndMeth=Round
  CAN3_AntiTheftSeatFold : Outport
  wires:
  Data Type Conversion/1 -> CAN3_AntiTheftSeatFold/1
  AntiTheftSeatFold/1 -> Data Type Conversion/1

== system halout/HAL_OUT/CAN3/FD_BCM1_0x216/AntitheftSta ==
  AntitheftSta : Inport
  Data Type Conversion : DataTypeConversion  OutDataTypeStr=uint8  RndMeth=Round
  CAN3_AntitheftSta : Outport
  wires:
  Data Type Conversion/1 -> CAN3_AntitheftSta/1
  AntitheftSta/1 -> Data Type Conversion/1

== system halout/HAL_OUT/CAN3/FD_BCM1_0x216/BCMBuzzerReq ==
  BCMBuzzerReq : Inport
  Data Type Conversion : DataTypeConversion  OutDataTypeStr=uint8  RndMeth=Round
  CAN3_BCM_Buzzer_Req : Outport
  wires:
  Data Type Conversion/1 -> CAN3_BCM_Buzzer_Req/1
  BCMBuzzerReq/1 -> Data Type Conversion/1

== system halout/HAL_OUT/CAN3/FD_BCM1_0x216/BCMDoorLockSta ==
  BCMDoorLockSta : Inport
  Data Type Conversion : DataTypeConversion  OutDataTypeStr=uint8  RndMeth=Round
  CAN3_BCM_DoorLock_Sta : Outport
  wires:
  Data Type Conversion/1 -> CAN3_BCM_DoorLock_Sta/1
  BCMDoorLockSta/1 -> Data Type Conversion/1

== system halout/HAL_OUT/CAN3/FD_BCM1_0x216/BrakeLamp ==
  BrakeLamp : Inport
  Data Type Conversion : DataTypeConversion  OutDataTypeStr=uint8  RndMeth=Round
  CAN3_BrakeLamp : Outport
  wires:
  Data Type Conversion/1 -> CAN3_BrakeLamp/1
  BrakeLamp/1 -> Data Type Conversion/1

== system halout/HAL_OUT/CAN3/FD_BCM1_0x216/CTDCtrl ==
  CTDCtrl : Inport
  Data Type Conversion : DataTypeConversion  OutDataTypeStr=uint8  RndMeth=Round
  CAN3_CTDCtrl : Outport
  wires:
  Data Type Conversion/1 -> CAN3_CTDCtrl/1
  CTDCtrl/1 -> Data Type Conversion/1

== system halout/HAL_OUT/CAN3/FD_BCM1_0x216/CTDLockSW ==
  CTDLockSW : Inport
  Data Type Conversion : DataTypeConversion  OutDataTypeStr=uint8  RndMeth=Round
  CAN3_CTDLockSW : Outport
  wires:
  Data Type Conversion/1 -> CAN3_CTDLockSW/1
  CTDLockSW/1 -> Data Type Conversion/1

== system halout/HAL_OUT/CAN3/FD_BCM1_0x216/CTDUnlockSW ==
  CTDUnlockSW : Inport
  Data Type Conversion : DataTypeConversion  OutDataTypeStr=uint8  RndMeth=Round
  CAN3_CTDUnlockSW : Outport
  wires:
  Data Type Conversion/1 -> CAN3_CTDUnlockSW/1
  CTDUnlockSW/1 -> Data Type Conversion/1

== system halout/HAL_OUT/CAN3/FD_BCM1_0x216/CrashDetd ==
  CrashDetd : Inport
  Data Type Conversion : DataTypeConversion  OutDataTypeStr=uint8  RndMeth=Round
  CAN3_CrashDetd : Outport
  wires:
  Data Type Conversion/1 -> CAN3_CrashDetd/1
  CrashDetd/1 -> Data Type Conversion/1

== system halout/HAL_OUT/CAN3/FD_BCM1_0x216/Dimmer ==
  Dimmer : Inport
  Data Type Conversion : DataTypeConversion  OutDataTypeStr=uint8  RndMeth=Round
  CAN3_Dimmer : Outport
  wires:
  Data Type Conversion/1 -> CAN3_Dimmer/1
  Dimmer/1 -> Data Type Conversion/1

== system halout/HAL_OUT/CAN3/FD_BCM1_0x216/DimmerEN ==
  DimmerEN : Inport
  Data Type Conversion : DataTypeConversion  OutDataTypeStr=uint8  RndMeth=Round
  CAN3_DimmerEN : Outport
  wires:
  Data Type Conversion/1 -> CAN3_DimmerEN/1
  DimmerEN/1 -> Data Type Conversion/1

== system halout/HAL_OUT/CAN3/FD_BCM1_0x216/DoorLockIND ==
  DoorLockIND : Inport
  Data Type Conversion : DataTypeConversion  OutDataTypeStr=uint8  RndMeth=Round
  CAN3_DoorLockIND : Outport
  wires:
  Data Type Conversion/1 -> CAN3_DoorLockIND/1
  DoorLockIND/1 -> Data Type Conversion/1

== system halout/HAL_OUT/CAN3/FD_BCM1_0x216/DrDoorSW ==
  DrDoorSW : Inport
  Data Type Conversion : DataTypeConversion  OutDataTypeStr=uint8  RndMeth=Round
  CAN3_DrDoorSW : Outport
  wires:
  Data Type Conversion/1 -> CAN3_DrDoorSW/1
  DrDoorSW/1 -> Data Type Conversion/1

== system halout/HAL_OUT/CAN3/FD_BCM1_0x216/FrChargingDoorCtrl ==
  FrChargingDoorCtrl : Inport
  Data Type Conversion : DataTypeConversion  OutDataTypeStr=uint8  RndMeth=Round
  CAN3_Fr_ChargingDoorCtrl : Outport
  wires:
  Data Type Conversion/1 -> CAN3_Fr_ChargingDoorCtrl/1
  FrChargingDoorCtrl/1 -> Data Type Conversion/1

== system halout/HAL_OUT/CAN3/FD_BCM1_0x216/FrFogLamp ==
  FrFogLamp : Inport
  Data Type Conversion : DataTypeConversion  OutDataTypeStr=uint8  RndMeth=Round
  CAN3_Fr_FogLamp : Outport
  wires:
  Data Type Conversion/1 -> CAN3_Fr_FogLamp/1
  FrFogLamp/1 -> Data Type Conversion/1

== system halout/HAL_OUT/CAN3/FD_BCM1_0x216/FrWiperH ==
  FrWiperH : Inport
  Data Type Conversion : DataTypeConversion  OutDataTypeStr=uint8  RndMeth=Round
  CAN3_Fr_Wiper_H : Outport
  wires:
  Data Type Conversion/1 -> CAN3_Fr_Wiper_H/1
  FrWiperH/1 -> Data Type Conversion/1

== system halout/HAL_OUT/CAN3/FD_BCM1_0x216/FrWiperL ==
  FrWiperL : Inport
  Data Type Conversion : DataTypeConversion  OutDataTypeStr=uint8  RndMeth=Round
  CAN3_Fr_Wiper_L : Outport
  wires:
  Data Type Conversion/1 -> CAN3_Fr_Wiper_L/1
  FrWiperL/1 -> Data Type Conversion/1

== system halout/HAL_OUT/CAN3/FD_BCM1_0x216/HBeam ==
  HBeam : Inport
  Data Type Conversion : DataTypeConversion  OutDataTypeStr=uint8  RndMeth=Round
  CAN3_H_Beam : Outport
  wires:
  Data Type Conversion/1 -> CAN3_H_Beam/1
  HBeam/1 -> Data Type Conversion/1

== system halout/HAL_OUT/CAN3/FD_BCM1_0x216/HazardSW ==
  HazardSW : Inport
  Data Type Conversion : DataTypeConversion  OutDataTypeStr=uint8  RndMeth=Round
  CAN3_HazardSW : Outport
  wires:
  Data Type Conversion/1 -> CAN3_HazardSW/1
  HazardSW/1 -> Data Type Conversion/1

== system halout/HAL_OUT/CAN3/FD_BCM1_0x216/HoodSW ==
  HoodSW : Inport
  Data Type Conversion : DataTypeConversion  OutDataTypeStr=uint8  RndMeth=Round
  CAN3_HoodSW : Outport
  wires:
  Data Type Conversion/1 -> CAN3_HoodSW/1
  HoodSW/1 -> Data Type Conversion/1

== system halout/HAL_OUT/CAN3/FD_BCM1_0x216/HornCtrl ==
  HornCtrl : Inport
  Data Type Conversion : DataTypeConversion  OutDataTypeStr=uint8  RndMeth=Round
  CAN3_HornCtrl : Outport
  wires:
  Data Type Conversion/1 -> CAN3_HornCtrl/1
  HornCtrl/1 -> Data Type Conversion/1

== system halout/HAL_OUT/CAN3/FD_BCM1_0x216/LAPMWdwEnable ==
  LAPMWdwEnable : Inport
  Data Type Conversion : DataTypeConversion  OutDataTypeStr=uint8  RndMeth=Round
  CAN3_L_APM_WdwEnable : Outport
  wires:
  Data Type Conversion/1 -> CAN3_L_APM_WdwEnable/1
  LAPMWdwEnable/1 -> Data Type Conversion/1

== system halout/HAL_OUT/CAN3/FD_BCM1_0x216/LBSD ==
  LBSD : Inport
  Data Type Conversion : DataTypeConversion  OutDataTypeStr=uint8  RndMeth=Round
  CAN3_LBSD : Outport
  wires:
  Data Type Conversion/1 -> CAN3_LBSD/1
  LBSD/1 -> Data Type Conversion/1

== system halout/HAL_OUT/CAN3/FD_BCM1_0x216/LBeam ==
  LBeam : Inport
  Data Type Conversion : DataTypeConversion  OutDataTypeStr=uint8  RndMeth=Round
  CAN3_L_Beam : Outport
  wires:
  Data Type Conversion/1 -> CAN3_L_Beam/1
  LBeam/1 -> Data Type Conversion/1

== system halout/HAL_OUT/CAN3/FD_BCM1_0x216/LDRL ==
  LDRL : Inport
  Data Type Conversion : DataTypeConversion  OutDataTypeStr=uint8  RndMeth=Round
  CAN3_LDRL : Outport
  wires:
  Data Type Conversion/1 -> CAN3_LDRL/1
  LDRL/1 -> Data Type Conversion/1

== system halout/HAL_OUT/CAN3/FD_BCM1_0x216/LTurnLP ==
  LTurnLP : Inport
  Data Type Conversion : DataTypeConversion  OutDataTypeStr=uint8  RndMeth=Round
  CAN3_LTurnLP : Outport
  wires:
  Data Type Conversion/1 -> CAN3_LTurnLP/1
  LTurnLP/1 -> Data Type Conversion/1

== system halout/HAL_OUT/CAN3/FD_BCM1_0x216/LockSetting ==
  LockSetting : Inport
  Data Type Conversion : DataTypeConversion  OutDataTypeStr=uint8  RndMeth=Round
  CAN3_LockSetting : Outport
  wires:
  Data Type Conversion/1 -> CAN3_LockSetting/1
  LockSetting/1 -> Data Type Conversion/1

== system halout/HAL_OUT/CAN3/FD_BCM1_0x216/MirrorCtrl ==
  MirrorCtrl : Inport
  Data Type Conversion : DataTypeConversion  OutDataTypeStr=uint8  RndMeth=Round
  CAN3_MirrorCtrl : Outport
  wires:
  Data Type Conversion/1 -> CAN3_MirrorCtrl/1
  MirrorCtrl/1 -> Data Type Conversion/1

== system halout/HAL_OUT/CAN3/FD_BCM1_0x216/MirrorDefog ==
  MirrorDefog : Inport
  Data Type Conversion : DataTypeConversion  OutDataTypeStr=uint8  RndMeth=Round
  CAN3_MirrorDefog : Outport
  wires:
  Data Type Conversion/1 -> CAN3_MirrorDefog/1
  MirrorDefog/1 -> Data Type Conversion/1

== system halout/HAL_OUT/CAN3/FD_BCM1_0x216/PmicBootReason ==
  PmicBootReason : Inport
  Data Type Conversion : DataTypeConversion  OutDataTypeStr=uint8  RndMeth=Round
  CAN3_PmicBootReason : Outport
  wires:
  Data Type Conversion/1 -> CAN3_PmicBootReason/1
  PmicBootReason/1 -> Data Type Conversion/1

== system halout/HAL_OUT/CAN3/FD_BCM1_0x216/PosLamp ==
  PosLamp : Inport
  Data Type Conversion : DataTypeConversion  OutDataTypeStr=uint8  RndMeth=Round
  CAN3_PosLamp : Outport
  wires:
  Data Type Conversion/1 -> CAN3_PosLamp/1
  PosLamp/1 -> Data Type Conversion/1

== system halout/HAL_OUT/CAN3/FD_BCM1_0x216/PsDoorSW ==
  PsDoorSW : Inport
  Data Type Conversion : DataTypeConversion  OutDataTypeStr=uint8  RndMeth=Round
  CAN3_PsDoorSW : Outport
  wires:
  Data Type Conversion/1 -> CAN3_PsDoorSW/1
  PsDoorSW/1 -> Data Type Conversion/1

== system halout/HAL_OUT/CAN3/FD_BCM1_0x216/RBSD ==
  RBSD : Inport
  Data Type Conversion : DataTypeConversion  OutDataTypeStr=uint8  RndMeth=Round
  CAN3_RBSD : Outport
  wires:
  Data Type Conversion/1 -> CAN3_RBSD/1
  RBSD/1 -> Data Type Conversion/1

== system halout/HAL_OUT/CAN3/FD_BCM1_0x216/RDRL ==
  RDRL : Inport
  Data Type Conversion : DataTypeConversion  OutDataTypeStr=uint8  RndMeth=Round
  CAN3_RDRL : Outport
  wires:
  Data Type Conversion/1 -> CAN3_RDRL/1
  RDRL/1 -> Data Type Conversion/1

== system halout/HAL_OUT/CAN3/FD_BCM1_0x216/RLDoorSW ==
  RLDoorSW : Inport
  Data Type Conversion : DataTypeConversion  OutDataTypeStr=uint8  RndMeth=Round
  CAN3_RLDoorSW : Outport
  wires:
  Data Type Conversion/1 -> CAN3_RLDoorSW/1
  RLDoorSW/1 -> Data Type Conversion/1

== system halout/HAL_OUT/CAN3/FD_BCM1_0x216/RRDoorSW ==
  RRDoorSW : Inport
  Data Type Conversion : DataTypeConversion  OutDataTypeStr=uint8  RndMeth=Round
  CAN3_RRDoorSW : Outport
  wires:
  Data Type Conversion/1 -> CAN3_RRDoorSW/1
  RRDoorSW/1 -> Data Type Conversion/1

== system halout/HAL_OUT/CAN3/FD_BCM1_0x216/RTurnLP ==
  RTurnLP : Inport
  Data Type Conversion : DataTypeConversion  OutDataTypeStr=uint8  RndMeth=Round
  CAN3_RTurnLP : Outport
  wires:
  Data Type Conversion/1 -> CAN3_RTurnLP/1
  RTurnLP/1 -> Data Type Conversion/1

== system halout/HAL_OUT/CAN3/FD_BCM1_0x216/ReverseLamp ==
  ReverseLamp : Inport
  Data Type Conversion : DataTypeConversion  OutDataTypeStr=uint8  RndMeth=Round
  CAN3_ReverseLamp : Outport
  wires:
  Data Type Conversion/1 -> CAN3_ReverseLamp/1
  ReverseLamp/1 -> Data Type Conversion/1

== system halout/HAL_OUT/CAN3/FD_BCM1_0x216/RoomLampH ==
  RoomLampH : Inport
  Data Type Conversion : DataTypeConversion  OutDataTypeStr=uint8  RndMeth=Round
  CAN3_RoomLampH : Outport
  wires:
  Data Type Conversion/1 -> CAN3_RoomLampH/1
  RoomLampH/1 -> Data Type Conversion/1

== system halout/HAL_OUT/CAN3/FD_BCM1_0x216/RoomLampL ==
  RoomLampL : Inport
  Data Type Conversion : DataTypeConversion  OutDataTypeStr=uint8  RndMeth=Round
  CAN3_RoomLampL : Outport
  wires:
  Data Type Conversion/1 -> CAN3_RoomLampL/1
  RoomLampL/1 -> Data Type Conversion/1

== system halout/HAL_OUT/CAN3/FD_BCM1_0x216/RrChargingDoorCtrl ==
  RrChargingDoorCtrl : Inport
  Data Type Conversion : DataTypeConversion  OutDataTypeStr=uint8  RndMeth=Round
  CAN3_Rr_ChargingDoorCtrl : Outport
  wires:
  Data Type Conversion/1 -> CAN3_Rr_ChargingDoorCtrl/1
  RrChargingDoorCtrl/1 -> Data Type Conversion/1

== system halout/HAL_OUT/CAN3/FD_BCM1_0x216/RrDefog ==
  RrDefog : Inport
  Data Type Conversion : DataTypeConversion  OutDataTypeStr=uint8  RndMeth=Round
  CAN3_Rr_Defog : Outport
  wires:
  Data Type Conversion/1 -> CAN3_Rr_Defog/1
  RrDefog/1 -> Data Type Conversion/1

== system halout/HAL_OUT/CAN3/FD_BCM1_0x216/RrFogLamp ==
  RrFogLamp : Inport
  Data Type Conversion : DataTypeConversion  OutDataTypeStr=uint8  RndMeth=Round
  CAN3_Rr_FogLamp : Outport
  wires:
  Data Type Conversion/1 -> CAN3_Rr_FogLamp/1
  RrFogLamp/1 -> Data Type Conversion/1

== system halout/HAL_OUT/CAN3/FD_BCM1_0x216/RrWiper ==
  RrWiper : Inport
  Data Type Conversion : DataTypeConversion  OutDataTypeStr=uint8  RndMeth=Round
  CAN3_Rr_Wiper : Outport
  wires:
  Data Type Conversion/1 -> CAN3_Rr_Wiper/1
  RrWiper/1 -> Data Type Conversion/1

== system halout/HAL_OUT/CAN3/FD_BCM1_0x216/TailgateHDSW ==
  TailgateHDSW : Inport
  Data Type Conversion : DataTypeConversion  OutDataTypeStr=uint8  RndMeth=Round
  CAN3_TailgateHDSW : Outport
  wires:
  Data Type Conversion/1 -> CAN3_TailgateHDSW/1
  TailgateHDSW/1 -> Data Type Conversion/1

== system halout/HAL_OUT/CAN3/FD_BCM1_0x216/TailgateRemote ==
  TailgateRemote : Inport
  Data Type Conversion : DataTypeConversion  OutDataTypeStr=uint8  RndMeth=Round
  CAN3_TailgateRemote : Outport
  wires:
  Data Type Conversion/1 -> CAN3_TailgateRemote/1
  TailgateRemote/1 -> Data Type Conversion/1

== system halout/HAL_OUT/CAN3/FD_BCM1_0x216/TailgateSW ==
  TailgateSW : Inport
  Data Type Conversion : DataTypeConversion  OutDataTypeStr=uint8  RndMeth=Round
  CAN3_Tailgate_SW : Outport
  wires:
  Data Type Conversion/1 -> CAN3_Tailgate_SW/1
  TailgateSW/1 -> Data Type Conversion/1

== system halout/HAL_OUT/CAN3/FD_BCM1_0x216/TrunkRel ==
  TrunkRel : Inport
  Data Type Conversion : DataTypeConversion  OutDataTypeStr=uint8  RndMeth=Round
  CAN3_TrunkRel : Outport
  wires:
  Data Type Conversion/1 -> CAN3_TrunkRel/1
  TrunkRel/1 -> Data Type Conversion/1

== system halout/HAL_OUT/CAN3/FD_BCM1_0x216/WasherCtrl ==
  WasherCtrl : Inport
  Data Type Conversion : DataTypeConversion  OutDataTypeStr=uint8  RndMeth=Round
  CAN3_WasherCtrl : Outport
  wires:
  Data Type Conversion/1 -> CAN3_WasherCtrl/1
  WasherCtrl/1 -> Data Type Conversion/1

== system halout/HAL_OUT/CAN3/FD_BCM1_0x216/WiperFixMode ==
  WiperFixMode : Inport
  Data Type Conversion : DataTypeConversion  OutDataTypeStr=uint8  RndMeth=Round
  CAN3_WiperFixMode : Outport
  wires:
  Data Type Conversion/1 -> CAN3_WiperFixMode/1
  WiperFixMode/1 -> Data Type Conversion/1

== system halout/HAL_OUT/CAN3/FD_BCM1_0x216/WisrBootReason ==
  WisrBootReason : Inport
  Data Type Conversion : DataTypeConversion  OutDataTypeStr=uint32  RndMeth=Round
  CAN3_WisrBootReason : Outport
  wires:
  Data Type Conversion/1 -> CAN3_WisrBootReason/1
  WisrBootReason/1 -> Data Type Conversion/1

== system halout/HAL_OUT/CAN3/FD_THCM1_0x182/BatteryMode ==
  BatteryMode : Inport
  Data Type Conversion : DataTypeConversion  OutDataTypeStr=uint8  RndMeth=Round
  CAN3_BatteryMode : Outport
  wires:
  Data Type Conversion/1 -> CAN3_BatteryMode/1
  BatteryMode/1 -> Data Type Conversion/1

== system halout/HAL_OUT/CAN3/FD_THCM1_0x182/CCUACLampSts ==
  CCUACLampSts : Inport
  Data Type Conversion : DataTypeConversion  OutDataTypeStr=uint8  RndMeth=Round
  CAN3_CCU_ACLampSts : Outport
  wires:
  Data Type Conversion/1 -> CAN3_CCU_ACLampSts/1
  CCUACLampSts/1 -> Data Type Conversion/1

== system halout/HAL_OUT/CAN3/FD_THCM1_0x182/CCUACMaxLampSts ==
  CCUACMaxLampSts : Inport
  Data Type Conversion : DataTypeConversion  OutDataTypeStr=uint8  RndMeth=Round
  CAN3_CCU_ACMaxLampSts : Outport
  wires:
  Data Type Conversion/1 -> CAN3_CCU_ACMaxLampSts/1
  CCUACMaxLampSts/1 -> Data Type Conversion/1

== system halout/HAL_OUT/CAN3/FD_THCM1_0x182/CCUAutoLampSts ==
  CCUAutoLampSts : Inport
  Data Type Conversion : DataTypeConversion  OutDataTypeStr=uint8  RndMeth=Round
  CAN3_CCU_AutoLampSts : Outport
  wires:
  Data Type Conversion/1 -> CAN3_CCU_AutoLampSts/1
  CCUAutoLampSts/1 -> Data Type Conversion/1

== system halout/HAL_OUT/CAN3/FD_THCM1_0x182/CCUAutoMidLampSts ==
  CCUAutoMidLampSts : Inport
  Data Type Conversion : DataTypeConversion  OutDataTypeStr=uint8  RndMeth=Round
  CAN3_CCU_AutoMidLampSts : Outport
  wires:
  Data Type Conversion/1 -> CAN3_CCU_AutoMidLampSts/1
  CCUAutoMidLampSts/1 -> Data Type Conversion/1

== system halout/HAL_OUT/CAN3/FD_THCM1_0x182/CCUDispalyRequest ==
  CCUDispalyRequest : Inport
  Data Type Conversion : DataTypeConversion  OutDataTypeStr=uint8  RndMeth=Round
  CAN3_CCU_Dispaly_Request : Outport
  wires:
  Data Type Conversion/1 -> CAN3_CCU_Dispaly_Request/1
  CCUDispalyRequest/1 -> Data Type Conversion/1

== system halout/HAL_OUT/CAN3/FD_THCM1_0x182/CCUEcoSts ==
  CCUEcoSts : Inport
  Data Type Conversion : DataTypeConversion  OutDataTypeStr=uint8  RndMeth=Round
  CAN3_CCU_EcoSts : Outport
  wires:
  Data Type Conversion/1 -> CAN3_CCU_EcoSts/1
  CCUEcoSts/1 -> Data Type Conversion/1

== system halout/HAL_OUT/CAN3/FD_THCM1_0x182/CCUFrtOnOffLampSts ==
  CCUFrtOnOffLampSts : Inport
  Data Type Conversion : DataTypeConversion  OutDataTypeStr=uint8  RndMeth=Round
  CAN3_CCU_FrtOnOffLampSts : Outport
  wires:
  Data Type Conversion/1 -> CAN3_CCU_FrtOnOffLampSts/1
  CCUFrtOnOffLampSts/1 -> Data Type Conversion/1

== system halout/HAL_OUT/CAN3/FD_THCM1_0x182/CCUHEATMaxLampSts ==
  CCUHEATMaxLampSts : Inport
  Data Type Conversion : DataTypeConversion  OutDataTypeStr=uint8  RndMeth=Round
  CAN3_CCU_HEATMaxLampSts : Outport
  wires:
  Data Type Conversion/1 -> CAN3_CCU_HEATMaxLampSts/1
  CCUHEATMaxLampSts/1 -> Data Type Conversion/1

== system halout/HAL_OUT/CAN3/FD_THCM1_0x182/CCURrOnOffLampSts ==
  CCURrOnOffLampSts : Inport
  Data Type Conversion : DataTypeConversion  OutDataTypeStr=uint8  RndMeth=Round
  CAN3_CCU_RrOnOffLampSts : Outport
  wires:
  Data Type Conversion/1 -> CAN3_CCU_RrOnOffLampSts/1
  CCURrOnOffLampSts/1 -> Data Type Conversion/1

== system halout/HAL_OUT/CAN3/FD_THCM1_0x182/CCUSyncLampSts ==
  CCUSyncLampSts : Inport
  Data Type Conversion : DataTypeConversion  OutDataTypeStr=uint8  RndMeth=Round
  CAN3_CCU_SyncLampSts : Outport
  wires:
  Data Type Conversion/1 -> CAN3_CCU_SyncLampSts/1
  CCUSyncLampSts/1 -> Data Type Conversion/1
